simulink model "DriveSimNull"  (R2015a)
settings: configuration reference "SIMULATION_CONFIGURATION" (kept outside this file)
settings Model: CovSFcnEnable=off  Creator=moritz  LastModifiedBy=moritz
settings ConfigSetRef: SourceLocation=Base Workspace

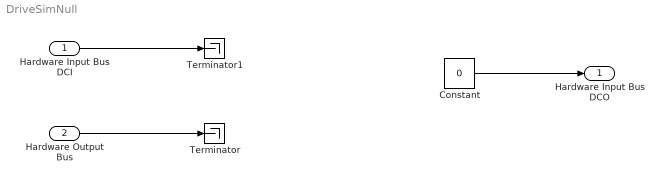
== system DriveSimNull ==
  Hardware Input Bus DCI : Inport  OutDataTypeStr=Bus: HARDWARE_INPUT_BUS  BusOutputAsStruct=on
  Hardware Output Bus : Inport  Port=2  OutDataTypeStr=Bus: HARDWARE_OUTPUT_BUS  BusOutputAsStruct=on
  Constant : Constant  Value=0  OutDataTypeStr=Bus: HARDWARE_INPUT_BUS  SampleTime=-1
  Terminator : Terminator
  Terminator1 : Terminator
  Hardware Input Bus DCO : Outport  OutDataTypeStr=Bus: HARDWARE_INPUT_BUS  BusOutputAsStruct=on
  wires:
  Hardware Output Bus/1 -> Terminator/1
  Hardware Input Bus DCI/1 -> Terminator1/1
  Constant/1 -> Hardware Input Bus DCO/1
